simulink model "model_discre"  (R2014b)
settings: Solver=ode45  StartTime=0.0  StopTime=10.0  RelTol=1e-3
values from neighbouring files (symbols this model uses):
  A = [ 0.9   -2.1     0.3     0.5     0.9 ... (first row only)    [HW8_main.m]
  B = [   1   -0.4 ... (first row only)    [HW8_main.m]
  C = [1  -2  -1   0   3 ... (first row only)    [HW8_main.m]
  Ed = inv(eye(r) + Kc*H)*Ec    [HW8_main.m]
  G_tilde = (eye(n)-Lo*C)*G    [HW8_main.m]
  H_tilde = (eye(n)-Lo*C)*H    [HW8_main.m]
  Kd = inv(eye(r) + Kc*H)*Kc*G    [HW8_main.m]
  Lo = (G-eye(n))/A*Ko/(eye(p)+C*(G-eye(n))/A*Ko)    [HW8_main.m]
  Ts = 0.02    [HW8_main.m]
  x_ini = [ 0.3 -0.2 0 -0.1 0.2]'    [HW8_main.m]
settings Model: Creator=123  LastModifiedBy=123

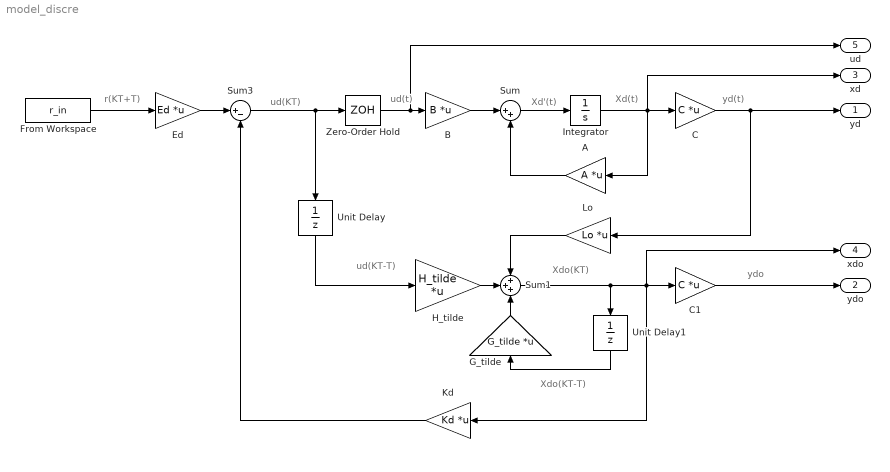
== system model_discre ==
  note: ud(t)
  note: ud(KT-T)
  note: ud(KT)
  note: r(KT+T)
  note: ydo
  note: yd(t)
  note: Xd(t)
  note: Xd'(t)
  note: Xdo(KT-T)
  note: Xdo(KT)
  A : Gain  Gain=A  Multiplication=Matrix(K*u)
  B : Gain  Gain=B  Multiplication=Matrix(K*u)
  C : Gain  Gain=C  Multiplication=Matrix(K*u)
  C1 : Gain  Gain=C  Multiplication=Matrix(K*u)
  Ed : Gain  Gain=Ed  Multiplication=Matrix(K*u)
  From Workspace : FromWorkspace  VariableName=r_in  SampleTime=Ts
  G_tilde : Gain  Gain=G_tilde  Multiplication=Matrix(K*u)
  H_tilde : Gain  Gain=H_tilde  Multiplication=Matrix(K*u)
  Integrator : Integrator  InitialCondition=x_ini
  Kd : Gain  Gain=Kd  Multiplication=Matrix(K*u)
  Lo : Gain  Gain=Lo  Multiplication=Matrix(K*u)
  Sum : Sum  Inputs=|++
  Sum1 : Sum  Inputs=+++
  Sum3 : Sum  Inputs=|+-
  Unit Delay : UnitDelay  SampleTime=Ts
  Unit Delay1 : UnitDelay  InitialCondition=pinv(C)*(C*x_ini)  SampleTime=Ts
  Zero-Order Hold : ZeroOrderHold  SampleTime=Ts
  yd : Outport
  ydo : Outport  Port=2
  xd : Outport  Port=3
  xdo : Outport  Port=4
  ud : Outport  Port=5
  wires:
  Integrator/1 -> xd/1, C/1, A/1
  B/1 -> Sum/1
  Sum/1 -> Integrator/1
  A/1 -> Sum/2
  Zero-Order Hold/1 -> ud/1, B/1
  C/1 -> Lo/1, yd/1
  Sum1/1 -> Unit Delay1/1, xdo/1, C1/1, Kd/1
  Unit Delay/1 -> H_tilde/1
  C1/1 -> ydo/1
  Sum3/1 -> Zero-Order Hold/1, Unit Delay/1
  H_tilde/1 -> Sum1/2
  Lo/1 -> Sum1/1
  G_tilde/1 -> Sum1/3
  Ed/1 -> Sum3/1
  From Workspace/1 -> Ed/1
  Kd/1 -> Sum3/2
  Unit Delay1/1 -> G_tilde/1
